simulink model "EKF2"  (R2019a)
settings: Solver=FixedStepDiscrete  StartTime=0.0  StopTime=10.0  FixedStep=Ts  RelTol=1e-3
values from neighbouring files (symbols this model uses):
  Ma = [1     Maxy     Maxz ... (first row only)    [IMU_init.m]
  Sa = diag([Sax;Say; Saz])    [IMU_init.m]
  Ts = 1e-3    (= 0.001)    [BARO_init.m]    (also in IMU_init.m)
undefined symbols (not defined in the file or in its folder): C, Jx, Jy, Jz, kb, m, Mo_pos, Mo_pqr, p0, R_air, So_pos, So_pqr, T0, V2
settings Model: Creator=david  LastModifiedBy=david

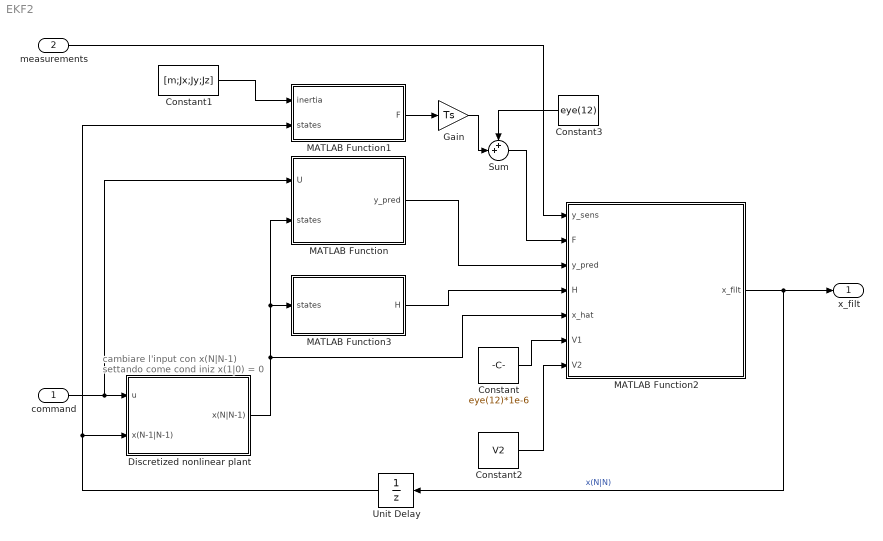
== system EKF2 ==
  note: cambiare l'input con x(N|N-1)
      | settando come cond iniz x(1|0) = 0
  command : Inport  PortDimensions=6
  measurements : Inport  Port=2  PortDimensions=16
  Constant : Constant  Value=eye(12)*1e-6
  Constant1 : Constant  Value=[m;Jx;Jy;Jz]
  Constant2 : Constant  Value=V2
  Constant3 : Constant  Value=eye(12)
  Discretized nonlinear plant : Subsystem
  Gain : Gain  Gain=Ts
  MATLAB Function : MATLAB Function  TreatAsAtomicUnit=on
  MATLAB Function1 : MATLAB Function  TreatAsAtomicUnit=on
  MATLAB Function2 : MATLAB Function  TreatAsAtomicUnit=on
  MATLAB Function3 : MATLAB Function  TreatAsAtomicUnit=on
  Sum : Sum  Inputs=++|
  Unit Delay : UnitDelay  InitialCondition=zeros(12,1)  SampleTime=-1  HasFrameUpgradeWarning=on
  x_filt : Outport
  wires:
  MATLAB Function3/1(H) -> MATLAB Function2/4(H)
  measurements/1 -> MATLAB Function2/1(y_sens)
  Constant1/1 -> MATLAB Function1/1(inertia)
  Constant/1 -> MATLAB Function2/6(V1)
  Constant2/1 -> MATLAB Function2/7(V2)
  MATLAB Function1/1(F) -> Gain/1
  Gain/1 -> Sum/2
  Discretized nonlinear plant/1(x(N|N-1)) -> MATLAB Function2/5(x_hat), MATLAB Function/2(states), MATLAB Function3/1(states)
  MATLAB Function2/1(x_filt) -> Unit Delay/1, x_filt/1  "x(N|N)"
  MATLAB Function/1(y_pred) -> MATLAB Function2/3(y_pred)
  Unit Delay/1 -> Discretized nonlinear plant/2(x(N-1|N-1)), MATLAB Function1/2(states)
  command/1 -> MATLAB Function/1(U), Discretized nonlinear plant/1(u)
  Sum/1 -> MATLAB Function2/2(F)
  Constant3/1 -> Sum/1

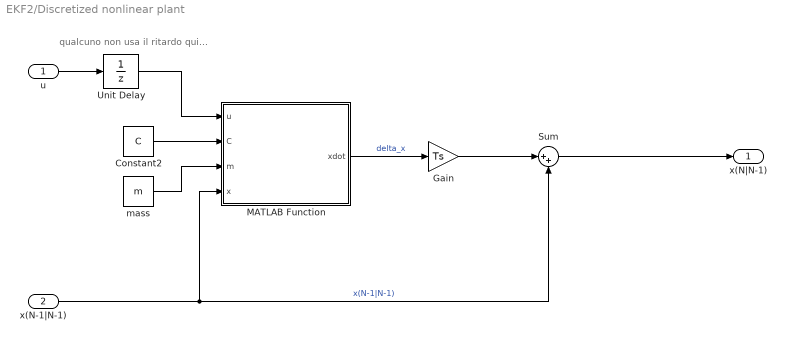
== system EKF2/Discretized nonlinear plant ==
  note: qualcuno non usa il ritardo qui...
  u : Inport
  x(N-1|N-1) : Inport  Port=2
  Constant2 : Constant  Value=C
  Gain : Gain  Gain=Ts
  MATLAB Function : MATLAB Function  TreatAsAtomicUnit=on
  Sum : Sum  Inputs=|++
  Unit Delay : UnitDelay  InitialCondition=zeros(6,1)  SampleTime=-1  HasFrameUpgradeWarning=on
  mass : Constant  Value=m
  x(N|N-1) : Outport
  wires:
  MATLAB Function/1(xdot) -> Gain/1  "delta_x"
  mass/1 -> MATLAB Function/3(m)
  Gain/1 -> Sum/1
  Sum/1 -> x(N|N-1)/1
  Constant2/1 -> MATLAB Function/2(C)
  x(N-1|N-1)/1 -> MATLAB Function/4(x), Sum/2  "x(N-1|N-1)"
  u/1 -> Unit Delay/1
  Unit Delay/1 -> MATLAB Function/1(u)

== matlab function EKF2/MATLAB Function1 ==
  data: inertia input; states input; F output
function F = jacobianF(inertia,states)

m = inertia(1);
Jx = inertia(2);
Jy = inertia(3);
Jz = inertia(4);

ph = states(4);
th = states(5);
ps = states(6);
u = states(7);
v = states(8);
w = states(9);
p = states(10);
q = states(11);
r = states(12);

F = zeros(12);
F(1,4) = v*(sin(ph)*sin(ps)) + w*(cos(ph)*sin(ps) - sin(ph)*sin(th)*cos(ps));
F(1,5) = -sin(th)*cos(ps)*u + sin(ph)*cos(th)*cos(ps)*v + ...
    cos(ph)*cos(th)*cos(ps)*w;
F(1,6) = -cos(th)*sin(ps)*u + v*(-cos(ph)*cos(ps) - ...
    sin(ph)*sin(th)*sin(ps)) + w*(sin(ph)*cos(ps) - cos(ph)*sin(th)*sin(ps));
F(1,7) = cos(th)*cos(ps);
F(1,8) = -cos(ph)*sin(ps) + sin(ph)*sin(th)*cos(ps);
F(1,9) = sin(ph)*sin(ps) + cos(ph)*sin(th)*cos(ps);
F(2,4) = v*(-sin(ph)*cos(ps) + cos(ph)*sin(th)*sin(ps)) + ...
    w*(-cos(ph)*cos(ps) - sin(ph)*sin(th)*sin(ps));
F(2,5) = -sin(th)*sin(ps)*u + v*sin(ph)*cos(th)*sin(ps) + w*cos(ph)*cos(th)*sin(ps);
F(2,6) = u*cos(th)*cos(ps) + v*(-cos(ph)*sin(ps) + ...
    sin(ph)*sin(th)*cos(ps)) + w*(sin(ph)*sin(ps) + cos(ph)*sin(th)*cos(ps));
F(2,7) = cos(th)*sin(ps);
F(2,8) = cos(ph)*cos(ps) + sin(ph)*sin(th)*sin(ps);
F(2,9) = -sin(ph)*cos(ps) + cos(ph)*sin(th)*sin(ps);
F(3,4) = cos(ph)*cos(th)*v - sin(ph)*cos(th)*w;
F(3,5) = -cos(th)*u - sin(ph)*sin(th)*v - cos(ph)*sin(th)*w;
F(3,7) = -sin(th);
F(3,8) = sin(ph)*cos(th);
F(3,9) = cos(ph)*cos(th);
F(4,4) = q*tan(th)*cos(ph) - r*tan(th)*sin(ph);
F(4,5) = 1/cos(th)^2*(q*sin(ph) + r*cos(ph));
F(4,10) = 1;
F(4,11) = tan(th)*sin(ph);
F(4,12) = tan(th)*cos(ph);
F(5,4) = -q*sin(ph) - r*cos(ph);
F(5,11) = cos(ph);
F(5,12) = -sin(ph);
F(6,4) = 1/cos(th)*(q*cos(ph) - r*sin(ph));
F(6,5) = 1/cos(th)^2*(q*sin(ph) + r*cos(ph));
F(6,11) = sin(ph)/cos(th);
F(6,12) = cos(ph)/cos(th);
F(7,5) = -9.81*cos(th);
F(7,8) = r;
F(7,9) = -q;
F(7,11) = -w;
F(7,12) = v;
F(8,4) = 9.81*cos(ph)*cos(th);
F(8,5) = -9.81*sin(ph)*sin(th);
F(8,7) = -r;
F(8,9) = p;
F(8,10) = w;
F(8,12) = -u;
F(9,4) = -9.81*sin(ph)*cos(th);
F(9,5) = -9.81*cos(ph)*sin(th);
F(9,7) = q;
F(9,8) = -p;
F(9,10) = -v;
F(9,11) = u;
F(10,10) = q*(Jx - Jy + Jz)/(Jx*Jz);
F(10,11) = (Jy - Jz)/Jx*r + p*(Jx - Jy + Jz)/(Jx*Jz);
F(10,12) = (Jy - Jz)/Jx*q;
F(11,10) = (Jz - Jx)/Jy*r;
F(11,12) = (Jz - Jx)/Jy*p;
F(12,10) = q*(Jx - Jy)/Jz;
F(12,11) = p*(Jx - Jy)/Jz - r*(Jx - Jy + Jz)/(Jx*Jz);
F(12,12) = -q*(Jx - Jy + Jz)/(Jx*Jz);

end

== matlab function EKF2/Discretized nonlinear plant/MATLAB Function ==
  data: u input; C input; m input; x input; xdot output
function xdot = quadrotor_dynamics(u,C,m,x)

ph = x(4);
th = x(5);
ps = x(6);
U = x(7);
V = x(8);
W = x(9);
p = x(10);
q = x(11);
r = x(12);
% Rotation from body to NED
% Rb_ned = [cos(th)*cos(ps), -cos(ph)*sin(ps) + sin(ph)*sin(th)*...
%                 cos(ps), sin(ph)*sin(ps) + cos(ph)*sin(th)*cos(ps)
%             cos(th)*sin(ps), cos(ph)*sin(th)*cos(ps), -sin(ph)*...
%                 cos(ps) + cos(ph)*sin(th)*sin(ps)
%             sin(th), -sin(ph)*cos(th), -cos(ph)*cos(th) ];
        
% Rb_ned = [ cos(ph)*cos(ps), cos(th)*sin(ph), -sin(th)
%             cos(ps)*sin(th)*sin(ps) - cos(ps)*sin(ph), cos(ps)*...
%                 cos(ph) + sin(ph)*sin(th)*sin(ps), cos(th)*sin(ps)
%             sin(ph)*sin(ps) + cos(ph)*cos(ps)*sin(th), cos(ps)*...
%                 sin(ph)*sin(th) - cos(ph)*sin(ps), cos(th)*cos(ps) ];
            
Rb_ned = [ cos(th)*cos(ps), cos(th)*sin(ps), -sin(th)
            -cos(ph)*sin(ps) + sin(ph)*sin(th)*cos(ps), cos(ph)...
                *cos(ps) + sin(ph)*sin(th)*sin(ps), sin(ph)*cos(th)
            sin(ph)*sin(ps) + cos(ph)*sin(th)*cos(ps), -sin(ph)...
            *cos(ps) + cos(ph)*sin(th)*sin(ps), cos(ph)*cos(th) ];
% Rb_ned = zeros(3,3);        
% Rb_ned(1,:) = [cos(ps)*cos(th) -sin(th)*cos(ph)+cos(ps)*sin(th)*sin(ph) sin(ps)*sin(ph)+cos(ps)*cos(ph)*sin(th)];
% Rb_ned(2,:) = [sin(ps)*cos(th) cos(ps)*cos(ph)+sin(ps)*sin(th)*sin(ps) -cos(ps)*sin(ph)+sin(th)*sin(ps)*cos(ph)];
% Rb_ned(3,:) = [-sin(th) cos(th)*sin(ph) cos(th)*cos(ph)];
% Constants linked to Inertia Moments
c1 = C(1);
c2 = C(2);
c3 = C(3);
c4 = C(4);
c5 = C(5);
c6 = C(6);
c7 = C(7);
c8 = C(8);
c9 = C(9);
% Non-linear plant in the form x_dot = f(x) + g(x)*u
f = [ Rb_ned'*x(7:9)
        p + tan(th)*(q*sin(ph) + r*cos(ph))
        q*cos(ph) - r*sin(ph)
        1/cos(th)*(q*sin(ph) + r*cos(ph))
        r*V - q*W - 9.81*sin(th)
        -r*U + p*W + 9.81*sin(ph)*cos(th)
        q*U - p*V + 9.81*cos(ph)*cos(th)
        (c1*r + c2*p)*q
        c5*p*r - c6*(p^2 - r^2) 
        (c8*p - c2*r)*q ];

g = zeros(12,6);
g(7:9,1:3) = diag([1/m,1/m,1/m]);
g(10,4) = c3;
g(10,6) = c4;
g(11,5) = c7;
g(12,4) = c4;
g(12,6) = c9;

xdot = f + g*u;
end

== matlab function EKF2/MATLAB Function2 ==
  data: y_sens input; F input; y_pred input; H input; x_filt output; x_hat input; V1 input; V2 input
function x_filt  = ...
    extendedKalmanFilter(y_sens,F,y_pred,H,x_hat,V1,V2)
% shamalayaaaa

persistent P_old

if isempty(P_old)
    P_old = eye(12);
end

% x_hat = x_old + Ts*delta_x;

% Filter gain
K = P_old*H'*inv(H*P_old*H' + V2);

% Innovation
err = y_sens - y_pred; %H*x_hat;
% Corrector
x_filt = x_hat + K*err; % x(N|N)
% Measurement update
P0 = (eye(12) - K*H)*P_old;

% Time update - forecast covariance
P = F*P0*F' + V1;
P_old = P;


end

== matlab function EKF2/MATLAB Function3 ==
  data: states input; H output; Ma parameter; Sa parameter; kb parameter; R_air parameter; T0 parameter; p0 parameter; Mo_pos parameter; So_pos parameter; Mo_pqr parameter; So_pqr parameter
function H = ...
    jacobianH(states, Ma, Sa, kb, R_air, T0, p0, Mo_pos, So_pos, Mo_pqr, So_pqr)

h = states(3);
ph = states(4);
th = states(5);
ps = states(6);
u = states(7);
v = states(8);
w = states(9);
p = states(10);
q = states(11);
r = states(12);

H = zeros(16,12);

H(1,5) = -9.81*cos(th);
H(1,8) = r;
H(1,9) = -q;
H(1,11) = w;
H(1,12) = v;
H(2,4) = 9.81*cos(ph)*cos(th);
H(2,5) = -9.81*sin(ph)*sin(th);
H(2,7) = -r;
H(2,9) = p;
H(2,10) = w;
H(2,12) = p;
H(3,4) = -9.81*sin(ph)*cos(th);
H(3,5) = -9.81*cos(ph)*sin(th);
H(3,7) = q;
H(3,8) = -p;
H(3,10) = -v;
H(3,11) = u;
% Add the misalignment factor...
H(4:6,10:12) = Ma*eye(3)*Sa;
H(7,3) = -(kb*p0*9.81)/(R_air*T0)*exp(-(9.81*h)/(R_air*T0));
H(8:10,1:3) = Mo_pos*eye(3)*So_pos;
H(11:13,10:12) = Mo_pqr*eye(3)*So_pqr;
H(14:16,4:6) = eye(3);


end

== matlab function EKF2/MATLAB Function ==
  data: U input; states input; y_pred output; kb parameter; R_air parameter; T0 parameter; p0 parameter; m parameter
function y_pred = ...
    obsDynamics(U, states, kb, R_air, T0, p0, m)

pn = states(1);
pe = states(2);
h = states(3);
ph = states(4);
th = states(5);
ps = states(6);
u = states(7);
v = states(8);
w = states(9);
p = states(10);
q = states(11);
r = states(12);

y_pred = [ r*v - q*w - 9.81*sin(th);
        -r*u + p*w + 9.81*sin(ph)*cos(th);
        q*u - p*v + 9.81*cos(ph)*cos(th) + U(3)/m;
        p;
        q;
        r;
        h;%kb*p0*exp(-9.81*h/(R_air*T0));
        pn;
        pe;
        h;
        p;
        q;
        r;
        ph;
        th;
        ps ];


end
